simulink model "dcmotor_ParamEst"  (R2026a)
settings: Solver=ode15s  StopTime=4  EnableMultiTasking=on
PreLoadFcn:
  | load dcmotor_ParamEst_Data;
  | load dcmotor_ParamEst_Param_Start;
undefined symbols (not defined in the file or in its folder): DC_Motor_B, DC_Motor_K, DC_Motor_R
libraries: fl_lib x20, nesl_utility x6
Description:
  | Copyright 2014-2026 The MathWorks, Inc.
settings Model: Creator=smiller  LastModifiedBy=smiller
settings DataIOCC: ExternalInput=[SS_DC_Motor_SPE_Input_time SS_DC_Motor_SPE_Input_Signal]  LoadExternalInput=on
settings OptimizationCC: InitFltsAndDblsToZero=on
settings DebuggingCC: SaveWithParameterizedLinksMsg=none  UnderspecifiedInitializationDetection=Classic
settings HardwareCC: ProdHWDeviceType=32-bit Generic
settings GRTTargetCC: TargetFcnLib=ansi_tfl_tmw.mat  CombineOutputUpdateFcns=off  GRTInterface=on
settings SimscapeCC: SimscapeNormalizeSystem=off  SimscapeNominalValues="[{\"value\":\"1\",\"unit\":\"A\"},{\"value\":\"1\",\"unit\":\"bar\"},{\"value\":\"1\",\"unit\":\"cm^2\"},{\"value\":\"1\",\"unit\":\"cm^3/s\"},{\"value\":\"1\",\"unit\":\"kJ/kg\"},{\"value\":\"1\",\"unit\":\"kW\"},{\"value\":\"1\",\"unit\":\"l\"},{\"value\":\"1\",\"unit\":\"N\"},{\"value\":\"1\",\"unit\":\"N*m\"},{\"value\":\"1\",\"unit\":\"V\"}]"  SimscapeLogName=simlog_motor_spe  SimscapeLogDataHistory=5000.0

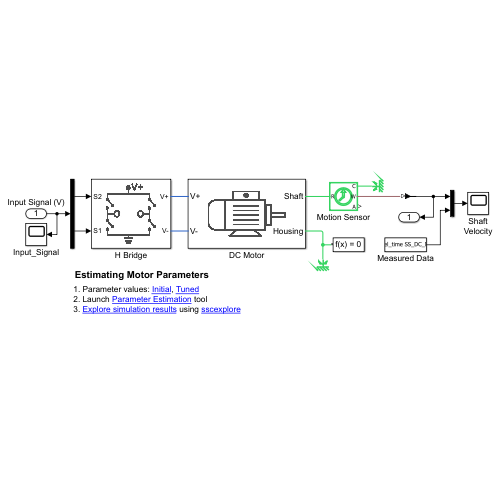
[thumbnail: Simulink's stored preview of the top-level diagram]
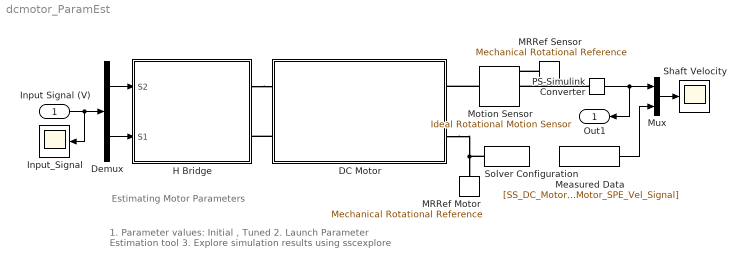
== system dcmotor_ParamEst ==
  note: 1. Parameter values: Initial , Tuned
      | 2. Launch Parameter Estimation tool
      | 3. Explore simulation results using sscexplore
  note: Estimating Motor Parameters
  Input Signal (V) : Inport  PortDimensions=2
  DC Motor : Subsystem
      mask Display:
      | image(imread('SN_Motor.jpg'));
      | port_label('lconn',1,'V+');
      | port_label('lconn',2,'V-');
      | port_label('rconn',1,'Shaft');
      | port_label('rconn',2,'Housing');
  Demux : Demux  Outputs=2
  H Bridge : Subsystem
      mask Display: image(imread('SN_H_Bridge.jpg'));
  Input_Signal : Scope
      settings: ActiveDisplayYMinimum=-0.5  ActiveDisplayYMaximum=1.5  DataLoggingVariableName=PWin_SPE_Input_Signal
  MRRef Motor : fl_lib/Mechanical/Rotational Elements/Mechanical Rotational Reference
  MRRef Sensor : fl_lib/Mechanical/Rotational Elements/Mechanical Rotational Reference
  Measured Data : FromWorkspace  VariableName=[SS_DC_Motor_SPE_Vel_time SS_DC_Motor_SPE_Vel_Signal]
  Motion Sensor : fl_lib/Mechanical/Mechanical Sensors/Ideal Rotational Motion Sensor  reference=foundation.enum.MeasurementReference.difference  acceleration_port=false  velocity_port=true  position_port=true  wrap_angle=simscape.enum.onoff.off  offset=0 rad
  Mux : Mux  Inputs=2
  PS-Simulink Converter : nesl_utility/PS-Simulink Converter  PhysicalDomain=network_engine_domain  SubClassName=ps_output  LeftPortType=input  RightPortType=output  PseudoPeriodic=off  Frequencies=[]  VectorFormat=1-D array  Unit=1  AffineConversion=off
  Shaft Velocity : Scope
      settings: ActiveDisplayYMinimum=-1.5  ActiveDisplayYMaximum=1.5  DataLoggingVariableName=SS_DC_Motor_SPE_DATA
  Solver Configuration : nesl_utility/Solver Configuration  PhysicalDomain=network_engine_domain  SubClassName=solver  LeftPortType=input  RightPortType=generic  Tones=[]  Harmonics=[]  SimulateNoise=off  Profile=off  UseLocalSampling=off  EnableSwitchedLinearOptims=on  FrequencyDomain=off  UseCCode=off  RelTol=0.001  AbsTol=1e-06  MinStep=1e-09  ToWorkspace=off  RevertToSquareIcSolve=off  NumHomotopyIterations=100  PhasorMode=off  PhasorModeNumHarmonics=1  ConsistencySolver=NEWTON_FTOL  CanonicalOrdering=UNORDERED  OptimizeIntermediates=UNOPTIMIZED  IndexReductionMethod=DerivativeReplacement  DoDC=off  ResidualTolerance=1e-9  ConsistencyTolSource=GLOBAL  ConsistencyAbsTol=0.001  ConsistencyRelTol=0.001  ConsistencyTolFactor=0.001  UseLocalSolver=off  LocalSolverChoice=NE_BACKWARD_EULER_ADVANCER  ResolveIndetEquations=on  FunctionEvalNumThread=1  LocalSolverSampleTime=.001  DoFixedCost=off  MaxNonlinIter=12  MaxModeIter=1  ComputeImpulses=off  ImpulseIterations=2  LinearAlgebra=Sparse  LinearAlgebraNumThread=0  EquationFormulation=NE_TIME_EF  DelaysMemoryBudget=1024  AutomaticFiltering=on  FilteringTimeConstant=0.001  PartitionStorageMethod=AS_NEEDED  PartitionMemoryBudget=1024  PartitionMethod=FAST  MultibodyUseLocalSolver=off  MultibodyLocalSolverChoice=ODE1  MultibodyLocalSolverSampleTime=0.001
  Out1 : Outport  VectorParamsAs1DForOutWhenUnconnected=off
  wires:
  Input Signal (V)/1 -> Demux/1, Input_Signal/1
  Demux/1 -> H Bridge/1(S2)
  Demux/2 -> H Bridge/2(S1)
  Mux/1 -> Shaft Velocity/1
  Measured Data/1 -> Mux/2
  PS-Simulink Converter/1 -> Out1/1, Mux/1
  connections:
  DC Motor/RConn2 -- Solver Configuration/RConn1 -- MRRef Motor/LConn1
  Motion Sensor/LConn1 -- DC Motor/RConn1
  MRRef Sensor/LConn1 -- Motion Sensor/RConn1
  PS-Simulink Converter/LConn1 -- Motion Sensor/RConn2
  H Bridge/RConn1 -- DC Motor/LConn1
  DC Motor/LConn2 -- H Bridge/RConn2

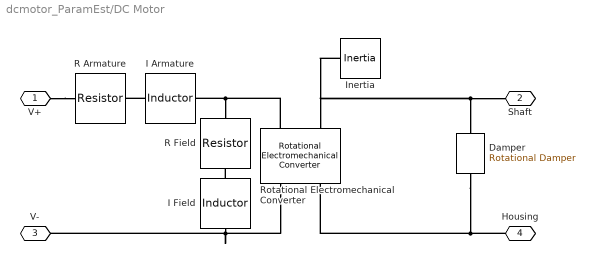
== system dcmotor_ParamEst/DC Motor ==
  " Damper" : fl_lib/Mechanical/Rotational Elements/Rotational Damper  D=DC_Motor_B N*m/(rad/s)  w_specify=off  w_priority=High  w=0 rad/s  w_nominal_specify=off  w_nominal_value=1  w_nominal_unit=rad/s  t_specify=off  t_priority=High  t=0 N*m  t_nominal_specify=off  t_nominal_value=1  t_nominal_unit=N*m
  I Armature : fl_lib/Electrical/Electrical Elements/Inductor  l=DC_Motor_L H  r=0 Ohm  g=1e-09 1/Ohm  i_specify=off  i_priority=High  i=0 A  i_nominal_specify=off  i_nominal_value=1  i_nominal_unit=A  v_specify=off  v_priority=High  v=0 V  v_nominal_specify=off  v_nominal_value=1  v_nominal_unit=V  i_L_specify=on  i_L_priority=High  i_L=0 A  i_L_nominal_specify=off  i_L_nominal_value=1  i_L_nominal_unit=A
  I Field : fl_lib/Electrical/Electrical Elements/Inductor  l=1e-6 H  r=0 Ohm  g=1e-09 1/Ohm  i_specify=off  i_priority=High  i=0 A  i_nominal_specify=off  i_nominal_value=1  i_nominal_unit=A  v_specify=off  v_priority=High  v=0 V  v_nominal_specify=off  v_nominal_value=1  v_nominal_unit=V  i_L_specify=on  i_L_priority=High  i_L=0 A  i_L_nominal_specify=off  i_L_nominal_value=1  i_L_nominal_unit=A
  Inertia : fl_lib/Mechanical/Rotational Elements/Inertia  inertia=DC_Motor_J kg*m^2  num_ports=foundation.enum.numPorts2.one  w_specify=on  w_priority=High  w=0 rad/s  w_nominal_specify=off  w_nominal_value=1  w_nominal_unit=rad/s  t_specify=off  t_priority=High  t=0 N*m  t_nominal_specify=off  t_nominal_value=1  t_nominal_unit=N*m
  R Armature : fl_lib/Electrical/Electrical Elements/Resistor  R=DC_Motor_R Ohm  i_specify=off  i_priority=High  i=0 A  i_nominal_specify=off  i_nominal_value=1  i_nominal_unit=A  v_specify=off  v_priority=High  v=0 V  v_nominal_specify=off  v_nominal_value=1  v_nominal_unit=V
  R Field : fl_lib/Electrical/Electrical Elements/Resistor  R=1e6 Ohm  i_specify=off  i_priority=High  i=0 A  i_nominal_specify=off  i_nominal_value=1  i_nominal_unit=A  v_specify=off  v_priority=High  v=0 V  v_nominal_specify=off  v_nominal_value=1  v_nominal_unit=V
  Rotational Electromechanical Converter : fl_lib/Electrical/Electrical Elements/Rotational Electromechanical Converter  K=DC_Motor_K V/(rad/s)  i_specify=off  i_priority=High  i=0 A  i_nominal_specify=off  i_nominal_value=1  i_nominal_unit=A  v_specify=off  v_priority=High  v=0 V  v_nominal_specify=off  v_nominal_value=1  v_nominal_unit=V  t_specify=off  t_priority=High  t=0 N*m  t_nominal_specify=off  t_nominal_value=1  t_nominal_unit=N*m  w_specify=off  w_priority=High  w=0 rad/s  w_nominal_specify=off  w_nominal_value=1  w_nominal_unit=rad/s
  V+ : PMIOPort  Side=Left
  Shaft : PMIOPort  Port=2  Side=Right
  V- : PMIOPort  Port=3  Side=Left
  Housing : PMIOPort  Port=4  Side=Right
  connections:
  I Armature/LConn1 -- R Armature/RConn1
  Rotational Electromechanical Converter/LConn1 -- R Field/LConn1 -- I Armature/RConn1
  Rotational Electromechanical Converter/RConn1 -- V-/RConn1 -- I Field/RConn1
  Inertia/LConn1 -- Rotational Electromechanical Converter/LConn2 -- " Damper"/LConn1 -- Shaft/RConn1
  V+/RConn1 -- R Armature/LConn1
  Housing/RConn1 -- " Damper"/RConn1 -- Rotational Electromechanical Converter/RConn2
  I Field/LConn1 -- R Field/RConn1

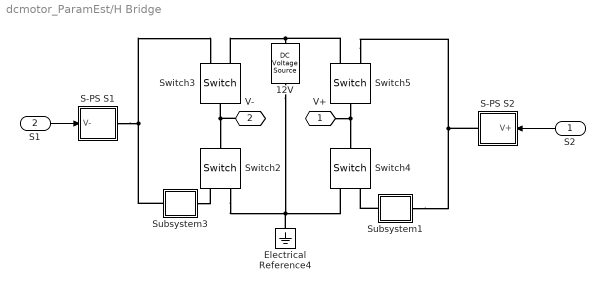
== system dcmotor_ParamEst/H Bridge ==
  S2 : Inport
  S1 : Inport  Port=2
  12V : fl_lib/Electrical/Electrical Sources/DC Voltage Source  v0=12 V
  Electrical Reference4 : fl_lib/Electrical/Electrical Elements/Electrical Reference
  S-PS S1 : Subsystem
  S-PS S2 : Subsystem
  Subsystem1 : Subsystem
      mask Display: disp('NOT');
  Subsystem3 : Subsystem
      mask Display: disp('NOT');
  Switch{2..5} (4 alike) : fl_lib/Electrical/Electrical Elements/Switch  R_closed=0.01 Ohm  G_open=1e-8 1/Ohm  Threshold=0  i_specify=off  i_priority=High  i=0 A  i_nominal_specify=off  i_nominal_value=1  i_nominal_unit=A  v_specify=off  v_priority=High  v=0 V  v_nominal_specify=off  v_nominal_value=1  v_nominal_unit=V
  V+ : PMIOPort  Side=Right
  V- : PMIOPort  Port=2  Side=Right
  wires:
  S2/1 -> S-PS S2/1(V+)
  S1/1 -> S-PS S1/1(V-)
  connections:
  Switch5/RConn1 -- Subsystem1/LConn1 -- S-PS S2/RConn1
  Subsystem1/RConn1 -- Switch4/RConn1
  Electrical Reference4/LConn1 -- 12V/RConn1 -- Switch4/RConn2 -- Switch2/RConn2
  Subsystem3/RConn1 -- Switch2/RConn1
  Switch3/LConn1 -- Switch2/LConn1 -- V-/RConn1
  S-PS S1/RConn1 -- Subsystem3/LConn1 -- Switch3/RConn1
  Switch5/RConn2 -- Switch3/RConn2 -- 12V/LConn1
  Switch5/LConn1 -- Switch4/LConn1 -- V+/RConn1

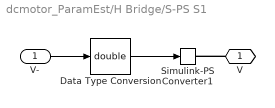
== system dcmotor_ParamEst/H Bridge/S-PS S1 ==
  V- : Inport
  Data Type Conversion : DataTypeConversion  OutDataTypeStr=double  SaturateOnIntegerOverflow=off  RndMeth=Floor
  Simulink-PS Converter1 : nesl_utility/Simulink-PS Converter  PhysicalDomain=network_engine_domain  SubClassName=ps_input  LeftPortType=input  RightPortType=output  PseudoPeriodic=off  Frequencies=[]  NoiseDistribution=none  NoiseParameters=[]  Unit=1  AffineConversion=off  FilteringAndDerivatives=zero  SimscapeFilterOrder=1  InputFilterTimeConstant=.001  UdotUserProvided=0
  V : PMIOPort  Side=Right
  wires:
  Data Type Conversion/1 -> Simulink-PS Converter1/1
  V-/1 -> Data Type Conversion/1
  connections:
  V/RConn1 -- Simulink-PS Converter1/RConn1

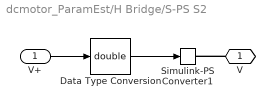
== system dcmotor_ParamEst/H Bridge/S-PS S2 ==
  V+ : Inport
  Data Type Conversion : DataTypeConversion  OutDataTypeStr=double  SaturateOnIntegerOverflow=off  RndMeth=Floor
  Simulink-PS Converter1 : nesl_utility/Simulink-PS Converter  PhysicalDomain=network_engine_domain  SubClassName=ps_input  LeftPortType=input  RightPortType=output  PseudoPeriodic=off  Frequencies=[]  NoiseDistribution=none  NoiseParameters=[]  Unit=1  AffineConversion=off  FilteringAndDerivatives=zero  SimscapeFilterOrder=1  InputFilterTimeConstant=.001  UdotUserProvided=0
  V : PMIOPort  Side=Right
  wires:
  V+/1 -> Data Type Conversion/1
  Data Type Conversion/1 -> Simulink-PS Converter1/1
  connections:
  V/RConn1 -- Simulink-PS Converter1/RConn1

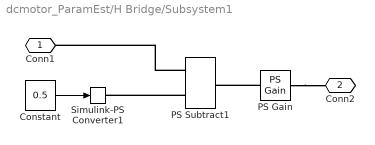
== system dcmotor_ParamEst/H Bridge/Subsystem1 ==
  Constant : Constant  Value=0.5
  PS Gain : fl_lib/Physical Signals/Functions/PS Gain  gain=-1
  PS Subtract1 : fl_lib/Physical Signals/Functions/PS Subtract
  Simulink-PS Converter1 : nesl_utility/Simulink-PS Converter  PhysicalDomain=network_engine_domain  SubClassName=ps_input  LeftPortType=input  RightPortType=output  PseudoPeriodic=off  Frequencies=[]  NoiseDistribution=none  NoiseParameters=[]  Unit=1  AffineConversion=off  FilteringAndDerivatives=zero  SimscapeFilterOrder=1  InputFilterTimeConstant=.001  UdotUserProvided=0
  Conn1 : PMIOPort  Side=Left
  Conn2 : PMIOPort  Port=2  Side=Right
  wires:
  Constant/1 -> Simulink-PS Converter1/1
  connections:
  PS Subtract1/LConn2 -- Simulink-PS Converter1/RConn1
  PS Subtract1/LConn1 -- Conn1/RConn1
  PS Gain/LConn1 -- PS Subtract1/RConn1
  PS Gain/RConn1 -- Conn2/RConn1

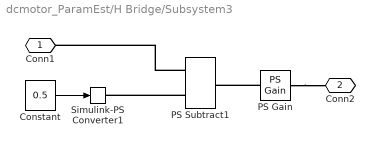
== system dcmotor_ParamEst/H Bridge/Subsystem3 ==
  Constant : Constant  Value=0.5
  PS Gain : fl_lib/Physical Signals/Functions/PS Gain  gain=-1
  PS Subtract1 : fl_lib/Physical Signals/Functions/PS Subtract
  Simulink-PS Converter1 : nesl_utility/Simulink-PS Converter  PhysicalDomain=network_engine_domain  SubClassName=ps_input  LeftPortType=input  RightPortType=output  PseudoPeriodic=off  Frequencies=[]  NoiseDistribution=none  NoiseParameters=[]  Unit=1  AffineConversion=off  FilteringAndDerivatives=zero  SimscapeFilterOrder=1  InputFilterTimeConstant=.001  UdotUserProvided=0
  Conn1 : PMIOPort  Side=Left
  Conn2 : PMIOPort  Port=2  Side=Right
  wires:
  Constant/1 -> Simulink-PS Converter1/1
  connections:
  PS Gain/RConn1 -- Conn2/RConn1
  PS Gain/LConn1 -- PS Subtract1/RConn1
  PS Subtract1/LConn1 -- Conn1/RConn1
  PS Subtract1/LConn2 -- Simulink-PS Converter1/RConn1
